simulink model "tm02"  (Simulink 8.1)
settings: Solver=ode45  StartTime=0.0  StopTime=1  RelTol=1e-3
values from neighbouring files (symbols this model uses):
  Fq = 1000*2*pi    (= 6283.18530718)    [pll1.m]    (also in temp02.m)
  st = 0.5e-5    (= 5e-06)    [pll1.m]    (also in temp02.m)
libraries: commanapbnd3 x2, commchan3 x1
settings Model: Creator=my88899  LastModifiedBy=my88899
settings DataIOCC: SignalLoggingSaveFormat=Dataset
settings OptimizationCC: ExpressionDepthLimit=128
settings DebuggingCC: FcnCallInpInsideContextMsg=EnableAllAsError
settings GRTTargetCC: CombineOutputUpdateFcns=on  GRTInterface=off

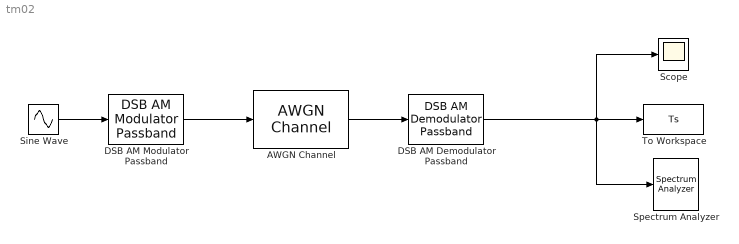
== system tm02 ==
  AWGN Channel : commchan3/AWGN Channel  InputProcessing=Columns as channels (frame based)  seed=2233  noiseMode="Signal to noise ratio  (Eb/No)"  EbNodB=40  EsNodB=10  SNRdB=10  bitsPerSym=1  Ps=1  Tsym=1  variance=1
  DSB AM Demodulator Passband : commanapbnd3/DSB AM Demodulator Passband  Fc=1e6  Ph=0  method=Butterworth  n=4  cf=1e4  Rp=0.1  Rs=50  Offset=1
  DSB AM Modulator Passband : commanapbnd3/DSB AM Modulator Passband  Fc=1e6  Ph=0  Offset=1
  Scope : Scope
      settings: TimeRange=500  YMin=-2  YMax=2
  Sine Wave : Sin  Frequency=Fq  Samples=spp  SampleTime=st
  Spectrum Analyzer : SpectrumAnalyzer
      settings: CopyFcn=scopeextensions.ScopeBlock.callback(gcbh, 'onBlockCopy', gcbh);  DeleteFcn=scopeextensions.ScopeBlock.callback(gcbh, 'onBlockDelete');  PreSaveFcn=scopeextensions.ScopeBlock.callback(gcbh, 'onModelSave');  NameChangeFcn=scopeextensions.ScopeBlock.callback(gcbh, 'onBlockRename');  CloseFcn=scopeextensions.ScopeBlock.callback(gcbh, 'onBlockClose');  PreDeleteFcn=scopeextensions.ScopeBlock.callback(gcbh, 'onBlockPreDelete');
  To Workspace : ToWorkspace  VariableName=Ts  SampleTime=-1  SaveFormat=Timeseries
  wires:
  DSB AM Demodulator Passband/1 -> Spectrum Analyzer/1, Scope/1, To Workspace/1
  Sine Wave/1 -> DSB AM Modulator Passband/1
  DSB AM Modulator Passband/1 -> AWGN Channel/1
  AWGN Channel/1 -> DSB AM Demodulator Passband/1
